simulink model "testing2"  (R2015a)
settings: Solver=ode3  StartTime=0.0  StopTime=30  FixedStep=0.01  RelTol=1e-3
values from neighbouring files (symbols this model uses):
  wheel_radius = 0.2538    [wrkspc_no_1.mat]    (also in wrkspc_no_10.mat; wrkspc_no_18.mat; wrkspc_no_22.mat)
libraries: simulink x1
settings Model: Creator=marco  LastModifiedBy=marco

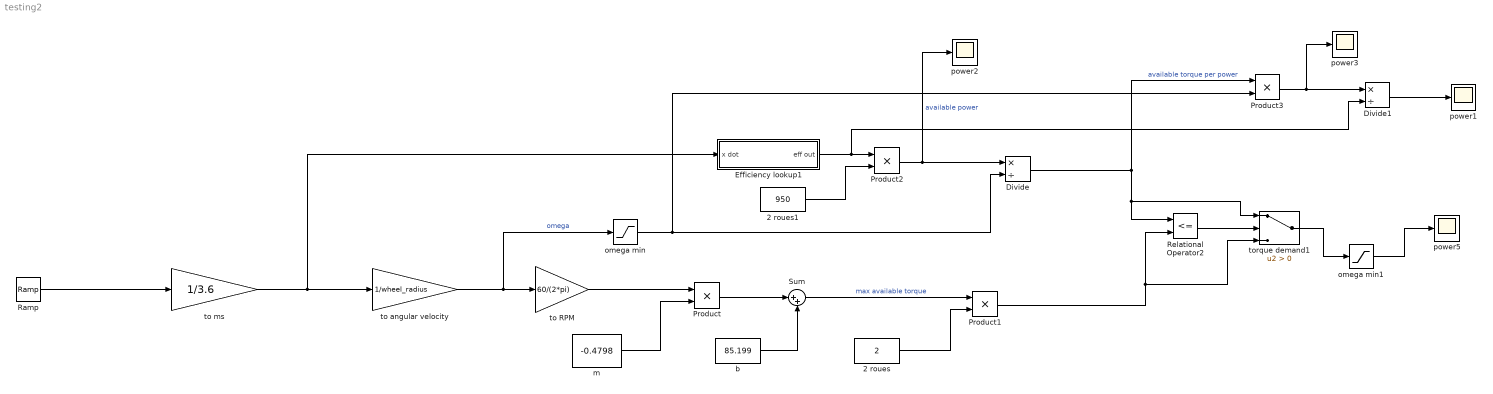
== system testing2 ==
  2 roues : Constant  Value=2
  2 roues1 : Constant  Value=950
  Divide : Product  Inputs=*/
  Divide1 : Product  Inputs=*/
  Efficiency lookup1 : Subsystem
  Product{,1..3} (4 alike) : Product
  Ramp : simulink/Sources/Ramp  slope=1  start=0  X0=0
  Relational Operator2 : RelationalOperator  Operator=<=  OutDataTypeStr=boolean
  Sum : Sum  Inputs=|++
  b : Constant  Value=85.199
  m : Constant  Value=-0.4798
  omega min : Saturate  UpperLimit=1000000  LowerLimit=0.1
  omega min1 : Saturate  UpperLimit=1000000  LowerLimit=0
  power{1..3,5} (4 alike) : Scope
      power1 settings: TimeRange=700  YMin=-500  YMax=1100  SaveName=ScopeData13  MaxDataPoints=100000
      power2 settings: TimeRange=700  YMin=-75  YMax=475  SaveName=ScopeData16  MaxDataPoints=scope_history
      power3 settings: TimeRange=700  YMin=-75  YMax=475  SaveName=ScopeData17  MaxDataPoints=scope_history
      power5 settings: TimeRange=700  YMin=-500  YMax=1100  MaxDataPoints=100000
  to RPM : Gain  Gain=60/(2*pi)
  to angular velocity : Gain  Gain=1/wheel_radius
  to ms : Gain  Gain=1/3.6
  torque demand1 : Switch  Criteria=u2 > Threshold
  wires:
  to ms/1 -> to angular velocity/1, Efficiency lookup1/1(x dot)
  Product1/1 -> torque demand1/3, Relational Operator2/2
  Product/1 -> Sum/1
  m/1 -> Product/2
  to angular velocity/1 -> omega min/1, to RPM/1  "omega"
  to RPM/1 -> Product/1
  b/1 -> Sum/2
  Sum/1 -> Product1/1  "max available torque"
  2 roues/1 -> Product1/2
  Relational Operator2/1 -> torque demand1/2
  Divide/1 -> Relational Operator2/1, torque demand1/1, Product3/1  "available torque per power"
  Product3/1 -> power3/1, Divide1/1
  Divide1/1 -> power1/1
  Efficiency lookup1/1(eff out) -> Divide1/2, Product2/1
  2 roues1/1 -> Product2/2
  Product2/1 -> power2/1, Divide/1  "available power"
  omega min/1 -> Product3/2, Divide/2
  Ramp/1 -> to ms/1
  torque demand1/1 -> omega min1/1
  omega min1/1 -> power5/1

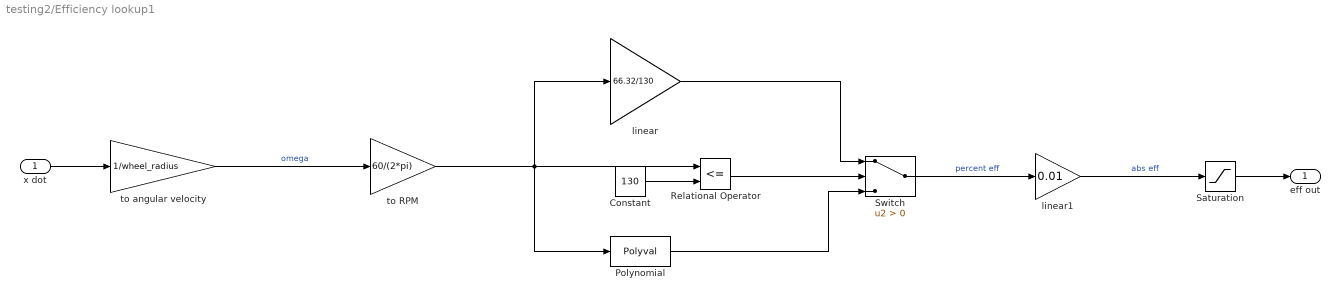
== system testing2/Efficiency lookup1 ==
  x dot : Inport
  Constant : Constant  Value=130
  Polynomial : Polyval  Coefs="[-0.000000281154604 0.00025333618 -0.0949601636 18.9528272 -2124.26186  126769.071 -3146791.96]"
  Relational Operator : RelationalOperator  Operator=<=  OutDataTypeStr=boolean
  Saturation : Saturate  UpperLimit=1  LowerLimit=0.05
  Switch : Switch  Criteria=u2 > Threshold
  linear : Gain  Gain=66.32/130
  linear1 : Gain  Gain=0.01
  to RPM : Gain  Gain=60/(2*pi)
  to angular velocity : Gain  Gain=1/wheel_radius
  eff out : Outport
  wires:
  x dot/1 -> to angular velocity/1
  to angular velocity/1 -> to RPM/1  "omega"
  Saturation/1 -> eff out/1
  Constant/1 -> Relational Operator/2
  Relational Operator/1 -> Switch/2
  Polynomial/1 -> Switch/3
  linear/1 -> Switch/1
  linear1/1 -> Saturation/1  "abs eff"
  to RPM/1 -> Polynomial/1, linear/1, Relational Operator/1
  Switch/1 -> linear1/1  "percent eff"
